simulink model "GFo_29bus"  (R2016b)
settings: Solver=ode1  StartTime=0.0  StopTime=4.5  FixedStep=Time_Step  RelTol=1e-3  EnableMultiTasking=on
PreLoadFcn:
  | Init_29bus;
InitFcn:
  | Init_29bus;
undefined symbols (not defined in the file): D1, D11, Delta, Time_Step, VSC01_Delta_P_Time_Step, VSC01_Delta_P_Value
libraries: powerlib x168, sps_avr x6, GFo_Lib x1
(part 1 of 4)
Description:
  | Copyright 2008-2017 The MathWorks, Inc.
settings Model: Creator=MathWorks  LastModifiedBy=Frederic_Colas
settings DataIOCC: SaveFormat=StructureWithTime  SignalLoggingSaveFormat=ModelDataLogs  SaveOutput=off  SignalLogging=off  DSMLogging=off  SaveTime=off
settings OptimizationCC: ExpressionDepthLimit=2147483647  LifeSpan=inf
settings DebuggingCC: UnderspecifiedInitializationDetection=Classic  MergeDetectMultiDrivingBlocksExec=none  SolverPrmCheckMsg=warning  FcnCallInpInsideContextMsg=warning  UnconnectedInputMsg=none  UnconnectedOutputMsg=none  UnconnectedLineMsg=none  StateNameClashWarn=warning  SFUnexpectedBacktrackingDiag=warning  SFNoUnconditionalDefaultTransitionDiag=warning  SFExecutionAtInitializationDiag=none
settings HardwareCC: ProdBitPerPointer=32  ProdBitPerSizeT=32  ProdBitPerPtrDiffT=32  ProdLargestAtomicFloat=None  ProdIntDivRoundTo=Undefined  ProdEndianess=Unspecified  ProdWordSize=32  ProdHWDeviceType=32-bit Generic
settings ModelReferenceCC: PropagateSignalLabelsOutOfModel=off
settings GRTTargetCC: TargetLangStandard=C89/C90 (ANSI)  GeneratePreprocessorConditionals=Disable all  CombineOutputUpdateFcns=off  GRTInterface=on
settings ConfigComp: CovMetricSettings=dw  CovHtmlReporting=on  CovSaveCumulativeToWorkspaceVar=on  CovSaveSingleToWorkspaceVar=on  CovExternalEMLEnable=off  CovSFcnEnable=off
settings SimscapeCC: SimscapeNormalizeSystem=off

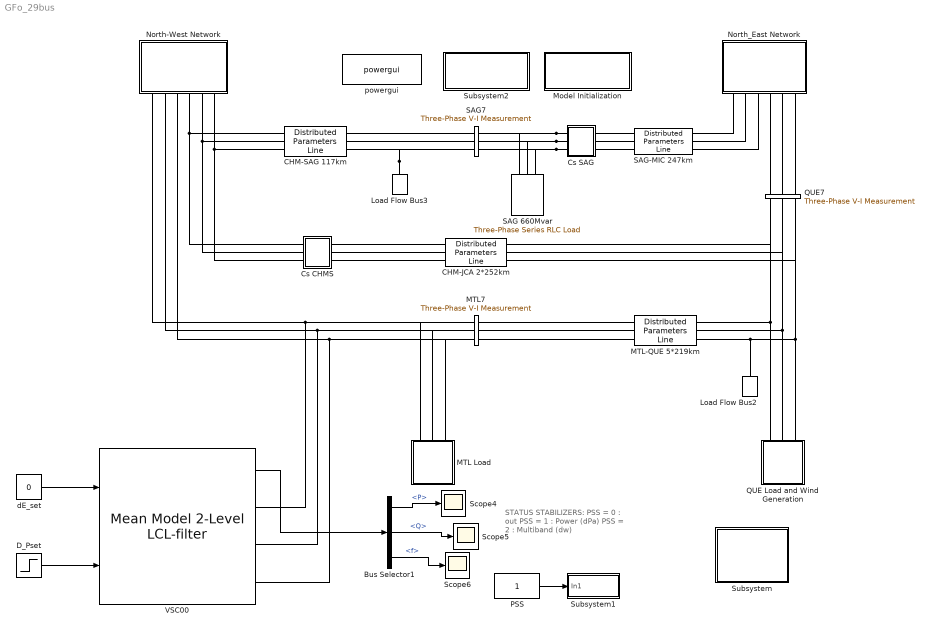
== system GFo_29bus ==
  note: STATUS STABILIZERS:
      | PSS = 0 :  out
      | PSS = 1 :  Power (dPa)
      | PSS = 2 :  Multiband (dw)
  Bus Selector1 : BusSelector  OutputSignals=control.P,control.Q,control.f
  CHM-JCA 2*252km : powerlib/Elements/Distributed Parameters Line  Phases=3  Frequency=60  Resistance="[0.01273  0.3864]/2"  Inductance="[0.9337e-3  4.1264e-3]/2"  Capacitance=[12.74e-9 7.751e-9]*2  Length=252  x1=[-0.00144 7.58185541586068e-08 0 0;-0.0014 7.65417383351047e-08 0 0;-0.00136 7.72475175803731e-08 0 0;-0.00132 7.7935731406298e-08 0 0;-0.00128 7.86062233189901e-08 0 0;-0.00124 7.92588408543707e-08 0 0;-0.0012 7.98934356128402e-08 0 0;-0.00116 8.0509863293023e-08 0 0;-0.00112 8.11079837245804e-08 0 0;-0.00108 8.16876609000843e-08 0 0;-0.00104 8.22487630059439e-08 0 0;-0.001 8.27911624523791e-08 0 0;-0.00096 8.33147359024331e-08 0 0;-0.00092 8.38193643000187e-08 0 0;-0.00088 8.43049328969899e-08 265107.476571619 -634085.697665156;-0.00084 8.4771331279235e-08 274638.71072506 -630016.083683103;-0.0008 8.52184533917841e-08 284107.494404066 -625803.209476646;-0.00076 8.56461975629245e-08 293511.674488884 -621448.033017052;-0.00072 8.60544665273205e-08 302849.112550059 -616951.54463389;-0.00068 8.64431674481302e-08 312117.6853347 -612314.766789841;-0.00064 8.68122119381164e-08 321315.285249284 -607538.753848202;-0.0006 8.71615160797445e-08 330439.820838908 -602624.591833129;-0.00056 8.7491000444265e-08 339489.217262864 -597573.398182686;-0.00052 8.78005901097747e-08 348461.416766445 -592386.32149475;-0.00048 8.80902146782535e-08 357354.379148857 -587064.541265828;-0.00044 8.83598082915721e-08 366166.082227143 -581609.267622851;-0.0004 8.86093096464677e-08 374894.522296013 -576021.741048002;-0.00036 8.88386620084838e-08 383537.714583465 -570303.232096638;-0.00032 8.90478132248713e-08 392093.693702109 -564455.041108381;-0.00028 8.9236715736447e-08 400560.514096078 -558478.497911428;-0.00024 8.94053265884089e-08 408936.250483427 -552374.961520165;-0.0002 8.95536074401033e-08 417218.998293933 -546145.81982613;-0.00016 8.96815245737432e-08 425406.87410217 -539792.489282428;-0.00012 8.97890489020757e-08 433498.016055789 -533316.414581635;-8e-05 8.98761559749955e-08 441490.584298885 -526719.068327291;-4e-05 8.99428259851056e-08 449382.761390363 -520001.950699042]  x2=[-0.00144 5.32803550600203e-08 0 0;-0.0014 5.36606177085858e-08 0 0;-0.00136 5.40286783954339e-08 0 0;-0.00132 5.43844534267383e-08 0 0;-0.00128 5.4727861902325e-08 0 0;-0.00124 5.50588257340681e-08 0 0;-0.0012 5.53772696636464e-08 0 0;-0.00116 5.56831212796564e-08 0 0;-0.00112 5.59763110340781e-08 0 0;-0.00108 5.62567722580899e-08 0 0;-0.00104 5.6524441177228e-08 0 0;-0.001 5.67792569258883e-08 0 0;-0.00096 5.70211615611672e-08 0 0;-0.00092 5.72501000760366e-08 0 0;-0.00088 5.74660204118525e-08 37391.1571539928 -657437.531518169;-0.00084 5.76688734701927e-08 47300.4110583682 -656799.004144863;-0.0008 5.78586131240209e-08 57198.9092571704 -656011.126342008;-0.00076 5.80351962281761e-08 67084.4009172698 -655074.077266222;-0.00072 5.81985826291833e-08 76954.6381631119 -653988.069994383;-0.00068 5.83487351743838e-08 86807.3765878642 -652753.351475181;-0.00064 5.84856197203837e-08 96640.3757637755 -651370.202472958;-0.0006 5.86092051408177e-08 106451.399751629 -649838.937503871;-0.00056 5.87194633334269e-08 116238.217609177 -648159.904764368;-0.00052 5.88163692264492e-08 125998.603898436 -646333.486052014;-0.00048 5.88999007843202e-08 135730.339191735 -644360.096678674;-0.00044 5.89700390126839e-08 145431.210576389 -642240.185376075;-0.0004 5.90267679627121e-08 155099.012157905 -639974.234193764;-0.00036 5.90700747347307e-08 164731.545561572 -637562.7583895;-0.00032 5.90999494811533e-08 174326.620432363 -635006.306312086;-0.00028 5.91163854087202e-08 183882.054932996 -632305.459276678;-0.00024 5.9119378780043e-08 193395.676240069 -629460.8314326;-0.0002 5.91089289144552e-08 202865.321038138 -626473.069623693;-0.00016 5.90850381881658e-08 212288.836011639 -623342.853241228;-0.00012 5.90477120337202e-08 221664.078334532 -620070.894069415;-8e-05 5.89969589387638e-08 230988.916157562 -616657.936123555;-4e-05 5.89327904441129e-08 240261.229093021 -613104.755480852]  x3=[-0.00144 2.36399872362907e-10 0 0;-0.0014 2.3698780301264e-10 0 0;-0.00136 2.37521844679663e-10 0 0;-0.00132 2.38001875927508e-10 0 0;-0.00128 2.38427787601207e-10 0 0;-0.00124 2.3879948285212e-10 0 0;-0.0012 2.39116877159951e-10 0 0;-0.00116 2.39379898351972e-10 0 0;-0.00112 2.39588486619432e-10 0 0;-0.00108 2.39742594531158e-10 0 0;-0.00104 2.3984218704434e-10 0 0;-0.001 2.39887241512498e-10 0 0;-0.00096 2.39877747690637e-10 0 0;-0.00092 2.39813707737568e-10 0 0;-0.00088 2.39695136215424e-10 455.571171588368 206.549514807623;-0.00084 2.39522060086348e-10 452.404295965122 213.395298242838;-0.0008 2.39294518706359e-10 449.134547506341 220.192557427475;-0.00076 2.39012563816404e-10 445.762669724628 226.939746723414;-0.00072 2.38676259530594e-10 442.289429355914 233.635331877992;-0.00068 2.38285682321623e-10 438.715616185106 240.277790372887;-0.00064 2.3784092100338e-10 435.0420428665 246.865611770318;-0.0006 2.37342076710754e-10 431.269544738988 253.397298056511;-0.00056 2.36789262876635e-10 427.398979636113 259.871363982331;-0.00052 2.36182605206121e-10 423.431227691001 266.286337401017;-0.00048 2.35522241647935e-10 419.367191136227 272.640759602933;-0.00044 2.34808322363056e-10 415.207794098658 278.93318564727;-0.0004 2.34041009690572e-10 410.95398238931 285.162184690607;-0.00036 2.33220478110768e-10 406.606723288283 291.32634031228;-0.00032 2.3234691420545e-10 402.167005324807 297.424250836457;-0.00028 2.31420516615516e-10 397.63583805246 303.454529650872;-0.00024 2.30441495995789e-10 393.014251819606 309.415805522124;-0.0002 2.29410074967115e-10 388.303297535099 315.306722907489;-0.00016 2.28326488065742e-10 383.504046429318 321.125942263154;-0.00012 2.27190981689987e-10 378.617589810576 326.872140348821;-8e-05 2.26003814044207e-10 373.64503881697 332.544010528597;-4e-05 2.24765255080087e-10 368.587524163715 338.140263068117]  x4=[-0.00144 2.98762369143109e-11 0 0;-0.0014 3.33610867134922e-11 0 0;-0.00136 3.68383504892487e-11 0 0;-0.00132 4.03072375417843e-11 0 0;-0.00128 4.37669590760978e-11 0 0;-0.00124 4.72167283813475e-11 0 0;-0.0012 5.0655761009743e-11 0 0;-0.00116 5.40832749549216e-11 0 0;-0.00112 5.74984908297697e-11 0 0;-0.00108 6.0900632043649e-11 0 0;-0.00104 6.42889249789862e-11 0 0;-0.001 6.76625991671874e-11 0 0;-0.00096 7.10208874638352e-11 0 0;-0.00092 7.43630262231319e-11 0 0;-0.00088 7.76882554715449e-11 191.292923698852 -10030.067654583;-0.00084 8.09958190806186e-11 342.515245147739 -10026.0432674796;-0.0008 8.42849649389116e-11 493.659681583605 -10019.7390445981;-0.00076 8.755494512302e-11 644.691864065019 -10011.1564194644;-0.00072 9.08050160676491e-11 795.57744917613 -10000.2973436934;-0.00068 9.40344387346936e-11 946.282126836066 -9987.16428654539;-0.00064 9.72424787812883e-11 1096.77162810075 -9971.76023436423;-0.0006 1.00428406726792e-10 1247.01173295536 -9954.08868989858;-0.00056 1.03591498118663e-10 1396.96827809566 -9934.15367150525;-0.00052 1.06731033697197e-10 1546.60716469647 -9911.95971223551;-0.00048 1.09846299559078e-10 1695.8943661654 -9887.51185880431;-0.00044 1.12936587319713e-10 1844.79593588023 -9860.81567044268;-0.0004 1.16001194274315e-10 1993.27801490809 -9831.87721763366;-0.00036 1.19039423557691e-10 2141.30683970465 -9800.70308073184;-0.00032 1.22050584302702e-10 2288.84874979171 -9767.30034846712;-0.00028 1.25033991797362e-10 2435.87019541126 -9731.67661633277;-0.00024 1.27988967640534e-10 2582.33774515442 -9693.83998485828;-0.0002 1.30914839896195e-10 2728.21809356346 -9653.79905776734;-0.00016 1.33810943246225e-10 2873.47806870518 -9611.56294002149;-0.00012 1.36676619141698e-10 3018.0846397139 -9567.14123574966;-8e-05 1.39511215952626e-10 3162.00492430239 -9520.54404606434;-4e-05 1.42314089116141e-10 3305.20619623907 -9471.78196676461]  x5=0.00142516474882927  V1=ones(3,3)  V2=ones(3,3)  I1=ones(3,3)  I2=ones(3,3)  nHarmo=1  Measurements=None
      settings: AttributesFormatString=\n
  CHM-SAG 117km : powerlib/Elements/Distributed Parameters Line  Phases=3  Frequency=60  Resistance="[0.01273  0.3864]"  Inductance="[0.9337e-3  4.1264e-3]"  Capacitance=[12.74e-9 7.751e-9]  Length=117  x1=[-0.00068 8.42693918023938e-08 0 0;-0.00064 8.46287304397579e-08 0 0;-0.0006 8.49688252336271e-08 0 0;-0.00056 8.52895988493781e-08 0 0;-0.00052 8.55909783458569e-08 0 0;-0.00048 8.5872895191965e-08 0 0;-0.00044 8.61352852822428e-08 290848.852660508 -619220.434969194;-0.0004 8.63780889514465e-08 300152.999076882 -614764.343999159;-0.00036 8.66012509881155e-08 309388.893289675 -610168.4609188;-0.00032 8.68047206471272e-08 318554.435136189 -605433.830792297;-0.00028 8.69884516612358e-08 327647.540451251 -600561.530233711;-0.00024 8.71524022515931e-08 336666.141541125 -595552.667162172;-0.0002 8.72965351372487e-08 345608.187653698 -590408.380549948;-0.00016 8.74208175436273e-08 354471.645444797 -585129.840163451;-0.00012 8.75252212099815e-08 363254.499440556 -579718.246297247;-8e-05 8.7609722395818e-08 371954.752495714 -574174.829501111;-4e-05 8.76743018862957e-08 380570.426247757 -568500.85030022]  x2=[-0.00068 5.85375290287409e-08 0 0;-0.00064 5.87422836781654e-08 0 0;-0.0006 5.89336808388534e-08 0 0;-0.00056 5.9111676988741e-08 0 0;-0.00052 5.92762316530388e-08 0 0;-0.00048 5.94273074134351e-08 0 0;-0.00044 5.95648699166049e-08 342746.554477027 -587488.694993711;-0.0004 5.96888878820212e-08 351566.310869505 -582253.6313362;-0.00036 5.97993331090682e-08 360306.12411467 -576886.168224064;-0.00032 5.98961804834537e-08 368964.006854359 -571387.526172128;-0.00028 5.99794079829199e-08 377537.9903607 -565758.955524177;-0.00024 6.00489966822511e-08 386026.124983782 -560001.736168637;-0.0002 6.01049307575773e-08 394426.480594989 -554117.177247541;-0.00016 6.01471974899721e-08 402737.147025899 -548106.616858843;-0.00012 6.0175787268345e-08 410956.234502632 -541971.421752141;-8e-05 6.0190693591627e-08 419081.874075575 -535712.987017895;-4e-05 6.01919130702487e-08 427112.218044361 -529332.735770193]  x3=[-0.00068 1.24684359191143e-10 0 0;-0.00064 1.23197676625095e-10 0 0;-0.0006 1.21682979969794e-10 0 0;-0.00056 1.20140613654197e-10 0 0;-0.00052 1.18570928399104e-10 0 0;-0.00048 1.16974281137405e-10 0 0;-0.00044 1.15351034932918e-10 1711.78655763124 -3591.74036566269;-0.0004 1.13701558897833e-10 1765.75158267616 -3565.52011206945;-0.00036 1.12026228108775e-10 1819.31509103836 -3538.48908995047;-0.00032 1.10325423521518e-10 1872.46490283797 -3510.65344592705;-0.00028 1.08599531884358e-10 1925.18893226613 -3482.01950958462;-0.00024 1.0684894565017e-10 1977.47519033321 -3452.59379203337;-0.0002 1.05074062887167e-10 2029.31178759503 -3422.38298442771;-0.00016 1.03275287188384e-10 2080.68693685638 -3391.39395644476;-0.00012 1.01453027579902e-10 2131.58895585138 -3359.63375472225;-8e-05 9.96076984278424e-11 2182.00626989986 -3327.10960125617;-4e-05 9.77397193441404e-11 2231.92741453938 -3293.82889175853]  x4=[-0.00068 5.36479088013724e-11 0 0;-0.00064 5.62282252514651e-11 0 0;-0.0006 5.87957558880272e-11 0 0;-0.00056 6.13499168767334e-11 0 0;-0.00052 6.38901274234009e-11 0 0;-0.00048 6.64158099060574e-11 0 0;-0.00044 6.89263900062868e-11 280.209360770516 -1025.16710784167;-0.0004 7.14212968398246e-11 295.636136449481 -1020.82529325836;-0.00036 7.38999630863721e-11 310.995687020474 -1016.25135180659;-0.00032 7.63618251185998e-11 326.284519854151 -1011.44632356119;-0.00028 7.88063231303119e-11 341.499158401772 -1006.41130114416;-0.00024 8.1232901263741e-11 356.636142985735 -1001.14742947617;-0.0002 8.36410077359454e-11 371.692031586282 -995.655905516244;-0.00016 8.603009496428e-11 386.663400624182 -989.937977989575;-0.00012 8.83996196909117e-11 401.546845739224 -983.994947103573;-8e-05 9.07490431063515e-11 416.338982564337 -977.828164252211;-4e-05 9.30778309719753e-11 431.036447495169 -971.439031708729]  x5=0.000661683633385019  V1=ones(3,3)  V2=ones(3,3)  I1=ones(3,3)  I2=ones(3,3)  nHarmo=1  Measurements=None
      settings: AttributesFormatString=\n
  Cs CHMS : Subsystem  mask{Xc=33/2}
      mask prompts: Xc "Condensator Reactance at  60Hz  (ohm):"
      mask help: Series Compensation
      mask init:
      | Cs=1/Xc/(2*pi*60);
      mask Display: disp('Cs')
  Cs SAG : Subsystem  mask{Xc=22}
      mask prompts: Xc "Condensator Reactance at  60Hz  (ohm):"
      mask help: Series Compensation
      mask init:
      | Cs=1/Xc/(2*pi*60);
      mask Display: disp('Cs')
  D_Pset : Step  Time=VSC01_Delta_P_Time_Step  After=VSC01_Delta_P_Value  SampleTime=0
  Load Flow Bus2 : powerlib/Measurements/Load Flow Bus  LConnTagsString=a  Phases=single  Connectors=on one side  ID=QUE7  Vbase=735e3  Vref=1  Vangle=0  VLF=1.016  VLFb=1  VLFc=1  angleLF=-12.43  angleLFb=0  angleLFc=0
      settings: AttributesFormatString=%<ID>\n%<Vbase>V\n%<VLF>pu\n%<angleLF>deg.
  Load Flow Bus3 : powerlib/Measurements/Load Flow Bus  LConnTagsString=a  Phases=single  Connectors=on one side  ID=SAG7  Vbase=735e3  Vref=1  Vangle=0  VLF=1.034  VLFb=1  VLFc=1  angleLF=2.23  angleLFb=0  angleLFc=0
      settings: AttributesFormatString=%<ID>\n%<Vbase>V\n%<VLF>pu\n%<angleLF>deg.
  MTL Load : Subsystem
  MTL-QUE 5*219km : powerlib/Elements/Distributed Parameters Line  Phases=3  Frequency=60  Resistance="[0.01273  0.3864]/5"  Inductance="[0.9337e-3  4.1264e-3]/5"  Capacitance=[12.74e-9 7.751e-9]*5  Length=219  x1=[-0.00124 3.13140205846512e-07 -185450.121801635 -635277.147887541;-0.0012 3.15795384732076e-07 -175849.670170163 -638001.383948039;-0.00116 3.18378754470456e-07 -166209.231840158 -640580.543995716;-0.00112 3.2088972762565e-07 -156530.99896416 -643014.041551821;-0.00108 3.23327733224018e-07 -146817.172288863 -645301.323259993;-0.00104 3.2569221688411e-07 -137069.960654684 -647441.869012097;-0.001 3.27982640942732e-07 -127291.580493494 -649435.192066489;-0.00096 3.30198484577206e-07 -117484.255324616 -651280.839158696;-0.00092 3.32339243923798e-07 -107650.215249218 -652978.390604485;-0.00088 3.34404432192293e-07 -97791.6964432079 -654527.460395296;-0.00084 3.36393579776688e-07 -87910.9406487465 -655927.696286018;-0.0008 3.38306234361977e-07 -78010.1946644932 -657178.779875083;-0.00076 3.40141961027001e-07 -68091.7098347044 -658280.426676874;-0.00072 3.41900342343347e-07 -58157.7415372972 -659232.386186407;-0.00068 3.43580978470266e-07 -48210.5486709954 -660034.441936299;-0.00064 3.45183487245598e-07 -38252.3931416758 -660686.411545989;-0.0006 3.46707504272665e-07 -28285.5393480304 -661188.146763211;-0.00056 3.4815268300314e-07 -18312.2536666614 -661539.533497702;-0.00052 3.4951869481584e-07 -8334.80393672679 -661740.49184715;-0.00048 3.50805229091459e-07 1644.54105574682 -661790.976115359;-0.00044 3.52011993283199e-07 11623.5120937662 -661690.974822642;-0.0004 3.53138712983289e-07 21599.8400453724 -661440.51070843;-0.00036 3.54185131985384e-07 31571.2563796214 -661039.640726103;-0.00032 3.55151012342829e-07 41535.4936824286 -660488.456030038;-0.00028 3.56036134422759e-07 51490.2861721592 -659787.081954881;-0.00024 3.56840296956046e-07 61433.3702148476 -658935.67798705;-0.0002 3.57563317083064e-07 71362.484838928 -657934.437728463;-0.00016 3.58205030395273e-07 81275.3722493598 -656783.588852522;-0.00012 3.58765290972599e-07 91169.7783410311 -655483.393052336;-8e-05 3.59243971416617e-07 101043.453211322 -654034.145981219;-4e-05 3.59640962879523e-07 110894.151671715 -652436.177185455]  x2=[-0.00124 5.50588257340681e-08 -51903.9427370369 -656450.777403812;-0.0012 5.53772696636464e-08 -41999.4092894903 -657158.855057256;-0.00116 5.56831212796564e-08 -32085.3255384587 -657717.500454157;-0.00112 5.59763110340782e-08 -22163.9458610917 -658126.586563369;-0.00108 5.62567722580899e-08 -12237.5262935698 -658386.020362239;-0.00104 5.6524441177228e-08 -2308.32401810053 -658495.742857757;-0.001 5.67792569258883e-08 7621.40315034427 -658455.729099975;-0.00096 5.70211615611672e-08 17549.3972774369 -658265.988187676;-0.00092 5.72501000760366e-08 27473.4008229281 -657926.563266307;-0.00088 5.74660204118525e-08 37391.1571539928 -657437.531518169;-0.00084 5.76688734701927e-08 47300.4110583682 -656799.004144863;-0.0008 5.78586131240209e-08 57198.9092571704 -656011.126342008;-0.00076 5.80351962281761e-08 67084.4009172698 -655074.077266222;-0.00072 5.81985826291833e-08 76954.6381631119 -653988.069994383;-0.00068 5.83487351743838e-08 86807.3765878643 -652753.351475181;-0.00064 5.84856197203837e-08 96640.3757637755 -651370.202472958;-0.0006 5.86092051408177e-08 106451.399751629 -649838.937503871;-0.00056 5.87194633334269e-08 116238.217609177 -648159.904764368;-0.00052 5.88163692264492e-08 125998.603898436 -646333.486052014;-0.00048 5.88999007843202e-08 135730.339191735 -644360.096678674;-0.00044 5.89700390126839e-08 145431.210576389 -642240.185376075;-0.0004 5.90267679627121e-08 155099.012157905 -639974.234193764;-0.00036 5.90700747347307e-08 164731.545561572 -637562.7583895;-0.00032 5.90999494811533e-08 174326.620432363 -635006.306312086;-0.00028 5.91163854087202e-08 183882.054932996 -632305.459276678;-0.00024 5.9119378780043e-08 193395.676240069 -629460.8314326;-0.0002 5.91089289144552e-08 202865.321038138 -626473.069623693;-0.00016 5.90850381881658e-08 212288.836011639 -623342.853241228;-0.00012 5.90477120337202e-08 221664.078334532 -620070.894069415;-8e-05 5.89969589387638e-08 230988.916157562 -616657.936123555;-4e-05 5.89327904441129e-08 240261.229093021 -613104.755480852]  x3=[-0.00124 2.99296411497035e-09 -6144.82838435572 -19926.8869416532;-0.0012 2.9563268208876e-09 -5843.65099570883 -20017.2814774563;-0.00116 2.91901728358006e-09 -5541.14481121902 -20103.1242560732;-0.00112 2.88104398691477e-09 -5237.37861818394 -20184.3957575961;-0.00108 2.84241556569193e-09 -4932.42149041631 -20261.0775015866;-0.00104 2.80314080368139e-09 -4626.34277253715 -20333.1520512774;-0.001 2.76322863162535e-09 -4319.2120642074 -20400.6030175373;-0.00096 2.72268812520754e-09 -4011.09920430154 -20463.4150625983;-0.00092 2.68152850298953e-09 -3702.07425502688 -20521.5739035431;-0.00088 2.63975912431445e-09 -3392.20748599195 -20575.0663155527;-0.00084 2.59738948717882e-09 -3081.56935822785 -20623.880134914;-0.0008 2.55442922607274e-09 -2770.23050816602 -20668.0042617853;-0.00076 2.51088810978911e-09 -2458.26173157608 -20707.4286627209;-0.00072 2.46677603920229e-09 -2145.73396746753 -20742.1443729517;-0.00068 2.42210304501672e-09 -1832.7182819588 -20772.1434984248;-0.00064 2.37687928548605e-09 -1519.28585211743 -20797.4192175977;-0.0006 2.33111504410318e-09 -1205.50794977506 -20817.9657829898;-0.00056 2.28482072726197e-09 -891.455925320772 -20833.7785224894;-0.00052 2.23800686189084e-09 -577.201191476651 -20844.8538404158;-0.00048 2.19068409305906e-09 -262.81520705916 -20851.1892183372;-0.00044 2.14286318155617e-09 51.6305392699954 -20852.7832156434;-0.0004 2.09455500144507e-09 366.064545259763 -20849.6354698731;-0.00036 2.0457705375893e-09 680.415311328745 -20841.7466967966;-0.00032 1.99652088315527e-09 994.611356823582 -20829.1186902527;-0.00028 1.94681723708966e-09 1308.58123627304 -20811.7543217414;-0.00024 1.89667090157298e-09 1622.25355563409 -20789.6575397702;-0.0002 1.84609327944948e-09 1935.55698852632 -20762.8333689569;-0.00016 1.79509587163426e-09 2248.42029245088 -20731.2879088865;-0.00012 1.74369027449807e-09 2560.77232499049 -20695.0283327246;-8e-05 1.69188817723041e-09 2872.54205998656 -20654.0628855862;-4e-05 1.63970135918147e-09 3183.65860368993 -20608.4008826607]  x4=[-0.00124 -9.87973508675663e-10 -1607.24957615672 -3120.54597153218;-0.0012 -9.24127780471541e-10 -1560.01251794718 -3144.42715530081;-0.00116 -8.60071913579479e-10 -1512.42072634402 -3167.59332345071;-0.00112 -7.95820473751212e-10 -1464.48502331026 -3190.03920819502;-0.00108 -7.31388071210079e-10 -1416.21630901138 -3211.75970553312;-0.00104 -6.66789357328774e-10 -1367.62555933676 -3232.74987641121;-0.001 -6.0203902129776e-10 -1318.72382340385 -3253.00494784545;-0.00096 -5.37151786785065e-10 -1269.52222104568 -3272.52031400727;-0.00092 -4.72142408588256e-10 -1220.03194028234 -3291.29153727071;-0.00088 -4.07025669279315e-10 -1170.26423477689 -3309.31434922145;-0.00084 -3.41816375843222e-10 -1120.23042127638 -3326.58465162749;-0.0008 -2.7652935631096e-10 -1069.94187703853 -3343.098517371;-0.00076 -2.1117945638776e-10 -1019.41003724462 -3358.85219134131;-0.00072 -1.45781536077312e-10 -968.646392399267 -3373.84209128882;-0.00068 -8.03504663027266e-11 -917.662485717529 -3388.06480863955;-0.00064 -1.49011255250167e-11 -866.469910500123 -3401.51710927021;-0.0006 5.05516036401357e-11 -815.080307497187 -3414.19593424366;-0.00056 1.15992837806559e-10 -763.50536226128 -3426.09840050444;-0.00052 1.81407696201944e-10 -711.756802490185 -3437.22180153436;-0.00048 2.46781304051607e-10 -659.846395360132 -3447.56360796794;-0.00044 3.1209879596088e-10 -607.785944850047 -3457.1214681676;-0.0004 3.77345319295376e-10 -555.587289057427 -3465.89320875834;-0.00036 4.42506037558352e-10 -503.262297506455 -3473.876835122;-0.00032 5.07566133764397e-10 -450.82286844898 -3481.07053185079;-0.00028 5.72510813808688e-10 -398.28092615895 -3487.47266316011;-0.00024 6.37325309831042e-10 -345.64841822094 -3493.08177326051;-0.0002 7.01994883573999e-10 -292.937312813372 -3497.89658668873;-0.00016 7.66504829734178e-10 -240.159595987053 -3501.91600859771;-0.00012 8.30840479306131e-10 -187.327268939656 -3505.13912500557;-8e-05 8.94987202917954e-10 -134.452345286743 -3507.56520300344;-4e-05 9.58930414157873e-10 -81.5468483299793 -3509.1936909221]  x5=0.00123853603172068  V1=ones(3,3)  V2=ones(3,3)  I1=ones(3,3)  I2=ones(3,3)  nHarmo=1  Measurements=None
      settings: AttributesFormatString=\n
  MTL7 : powerlib/Measurements/Three-Phase V-I Measurement  VoltageMeasurement=phase-to-ground  SetLabelV=on  LabelV=Vabc_MTL7  Vpu=on  VpuLL=off  CurrentMeasurement=no  SetLabelI=off  LabelI=A1  Ipu=off  Pbase=100e6  Vbase=735e3  OutputType=Magnitude  PhasorSimulation=off  PSBequivalent=0
  Model Initialization : Subsystem  mask(Model Functions){InitFcnX=Init_29bus;, prel=on, posl=off, inif=on, strf=off}
      mask prompts: InitFcnX "Initialisation"; prel "Preload Function"; posl "PostLoad Function"; inif "InitFcn"; strf "StartFcn"
      mask init:
      | currentBlock = gcb;
      | root = bdroot(currentBlock);
      | 
      | if ~strcmp(get_param(root,'BlockDiagramType'),'library')
      |     if prel==1
      |         set_param(root, 'PreLoadFcn', InitFcnX);
      |     else
      |         set_param(root, 'PreLoadFcn', '');
      |     end
      |     if inif==1
      |         set_param(root, 'InitFcn', InitFcnX);
      |     else
      |         set_param(root, 'InitFcn', '');
      |     end
      |     if strf==1
      |         set_param(root, 'StartFcn', InitFcnX);
      |     else
      |         set_param(root, 'StartFcn', '');
      |     end
      |     if posl==1
      |         set_param(root, 'PostLoadFcn', InitFcnX);
      |     else
      |         set_param(root, 'PostLoadFcn', '');
      |     end
      | end
      | 
      | pos = get_param(currentBlock, 'Position');
      | width = pos(3) - pos(1); height = pos(4) - pos(2);
      | txt = [ upper(root) '\n' '- InitFcn. . . . . '  get_param(root, 'InitFcn') ];
      settings: CopyFcn=set_param(gcb,'LinkStatus','none')
      mask Display:
      | %text(5, height*0.5, txt, 'horizontalAlignment', 'left', 'verticalAlignment', 'middle') ;
      | color('blue'),disp('Initialization Function\nParameters')
  North-West Network : Subsystem
  North_East Network : Subsystem
  PSS : Constant
  QUE Load and Wind Generation : Subsystem
  QUE7 : powerlib/Measurements/Three-Phase V-I Measurement  VoltageMeasurement=no  SetLabelV=on  LabelV=Vabc_QUE7  Vpu=on  VpuLL=off  CurrentMeasurement=no  SetLabelI=off  LabelI=A1  Ipu=off  Pbase=100e6  Vbase=735e3  OutputType=Magnitude  PhasorSimulation=off  PSBequivalent=0
  SAG 660Mvar : powerlib/Elements/Three-Phase Series RLC Load  LConnTagsString=A|B|C  Configuration=Y (grounded)  NominalVoltage=735e3  Vabc=[1e3 1e3 1e3]  Vabcp=[1e3 1e3 1e3]  NominalFrequency=60  UnbalancedPower=off  ActivePower=2200000  InductivePower=660e6  CapacitivePower=0  Pabc=[10e3 9e3 11e3]  QLabc=[100 90 110]  QCabc=[100 90 110]  Pabcp=[10e3 9e3 11e3]  QLabcp=[100 90 110]  QCabcp=[100 90 110]  Measurements=None  LoadType=constant Z
  SAG-MIC 247km : powerlib/Elements/Distributed Parameters Line  Phases=3  Frequency=60  Resistance="[0.01273  0.3864]/1"  Inductance="[0.9337e-3  4.1264e-3]/1"  Capacitance=[12.74e-9 7.751e-9]*1  Length=247  x1=[-0.0014 5.40873341776019e-08 78356.1362806858 -664124.955272439;-0.00136 5.45312309755495e-08 88361.5766055067 -662867.963935626;-0.00132 5.49627278418306e-08 98346.9242698054 -661460.242140145;-0.00128 5.53817266577788e-08 108309.908691633 -659902.10998979;-0.00124 5.57881321466767e-08 118248.264374249 -658193.921790378;-0.0012 5.61818518954209e-08 128159.731421276 -656336.065969173;-0.00116 5.65627963755356e-08 138042.056050579 -654328.964986568;-0.00112 5.69308789635314e-08 147892.991106762 -652173.075240017;-0.00108 5.72860159606018e-08 157710.296572141 -649868.886960258;-0.00104 5.76281266116564e-08 167491.740076115 -647416.924099835;-0.001 5.79571331236833e-08 177235.097402784 -644817.744213957;-0.00096 5.82729606834388e-08 186938.152996713 -642071.938333716;-0.00092 5.85755374744596e-08 196598.700466737 -639180.130831691;-0.00088 5.88647946933926e-08 206214.54308767 -636142.97927997;-0.00084 5.91406665656407e-08 215783.494299823 -632961.174300623;-0.0008 5.94030903603191e-08 225303.378206209 -629635.439408666;-0.00076 5.96520064045201e-08 234772.030067326 -626166.530847531;-0.00072 5.98873580968816e-08 244187.296793393 -622555.237417112;-0.00068 6.01090919204585e-08 253547.03743395 -618802.380294393;-0.00064 6.03171574548914e-08 262849.123664692 -614908.812846718;-0.0006 6.05115073878721e-08 272091.440271427 -610875.42043775;-0.00056 6.06920975259018e-08 281271.88563106 -606703.12022614;-0.00052 6.08588868043405e-08 290388.372189486 -602392.860956975;-0.00048 6.10118372967446e-08 299438.82693628 -597945.622746043;-0.00044 6.1150914223491e-08 308421.191876078 -593362.416856963;-0.0004 6.12760859596861e-08 317333.424496555 -588644.285471228;-0.00036 6.13873240423563e-08 326173.498232868 -583792.30145123;-0.00032 6.14846031769211e-08 334939.402928484 -578807.568096292;-0.00028 6.15679012429441e-08 343629.145292267 -573691.218891793;-0.00024 6.16371992991634e-08 352240.749351744 -568444.41725142;-0.0002 6.16924815877987e-08 360772.256902412 -563068.35625262;-0.00016 6.17337355381341e-08 369221.727953028 -557564.258365303;-0.00012 6.17609517693773e-08 377587.24116674 -551933.375173863;-8e-05 6.17741240927919e-08 385866.894297985 -546176.987092579;-4e-05 6.17732495131051e-08 394058.80462504 -540296.40307446]  x2=[-0.0014 1.88321190355134e-08 207429.358640792 -660594.51265032;-0.00136 1.89772310245538e-08 217366.870028888 -657391.600759257;-0.00132 1.9118027754912e-08 227254.95406523 -654039.203687286;-0.00128 1.92544772106255e-08 237091.362284782 -650538.08374059;-0.00124 1.93865483642649e-08 246873.857973139 -646889.037043652;-0.0012 1.95142111839887e-08 256600.216675142 -643092.893358225;-0.00116 1.96374366403727e-08 266268.226700699 -639150.515894644;-0.00112 1.97561967130107e-08 275875.689627704 -635062.801115549;-0.00108 1.98704643968863e-08 285420.420801939 -630830.678532028;-0.00104 1.99802137085137e-08 294900.249833843 -626455.110492261;-0.001 2.00854196918458e-08 304313.021092047 -621937.091962687;-0.00096 2.01860584239492e-08 313656.594193539 -617277.650301758;-0.00092 2.02821070204442e-08 322928.84449037 -612477.845026326;-0.00088 2.03735436407082e-08 332127.663552784 -607538.767570718;-0.00084 2.04603474928422e-08 341250.959648653 -602461.541038557;-0.0008 2.05424988383989e-08 350296.65821912 -597247.31994737;-0.00076 2.06199789968707e-08 359262.702350339 -591897.289966069;-0.00072 2.06927703499377e-08 368147.053241192 -586412.667645334;-0.00068 2.0760856345474e-08 376947.690666903 -580794.700140985;-0.00064 2.08242215013114e-08 385662.613438416 -575044.664930383;-0.0006 2.08828514087598e-08 394289.839857445 -569163.86952195;-0.00056 2.09367327358838e-08 402827.408167101 -563153.651157848;-0.00052 2.09858532305345e-08 411273.376997975 -557015.376509903;-0.00048 2.10302017231348e-08 419625.825809591 -550750.441368836;-0.00044 2.106976812922e-08 427882.855327117 -544360.270326871;-0.0004 2.11045434517305e-08 436042.587973246 -537846.316453797;-0.00036 2.1134519783058e-08 444103.168295141 -531210.06096655;-0.00032 2.11596903068431e-08 452062.763386348 -524453.0128924;-0.00028 2.11800492995259e-08 459919.563303584 -517576.708725808;-0.00024 2.11955921316469e-08 467671.781478303 -510582.712079043;-0.0002 2.12063152689001e-08 475317.655122943 -503472.61332663;-0.00016 2.12122162729367e-08 482855.445631773 -496248.029243709;-0.00012 2.12132938019192e-08 490283.438976234 -488910.602638398;-8e-05 2.12095476108268e-08 497599.946094697 -481462.001978234;-4e-05 2.12009785515111e-08 504803.303276536 -473903.92101077]  x3=[-0.0014 8.54566736572813e-11 -14.0413794849774 -3976.64390507056;-0.00136 8.48160555079537e-11 45.9239992686561 -3976.40393558055;-0.00132 8.4156150919026e-11 105.878935300888 -3975.25976612663;-0.00128 8.34771099471111e-11 165.809795376294 -3973.21165688308;-0.00124 8.27790870002702e-11 225.702951734113 -3970.26007357226;-0.0012 8.20622408029018e-11 285.544785187088 -3966.40568735879;-0.00116 8.13267343596495e-11 345.321688218344 -3961.64937469683;-0.00112 8.05727349183357e-11 405.020068075627 -3955.99221713087;-0.00108 7.98004139319312e-11 464.626349862174 -3949.43550104977;-0.00104 7.90099470195679e-11 524.126979623529 -3941.98071739421;-0.001 7.82015139266052e-11 583.508427429597 -3933.6295613177;-0.00096 7.73752984837567e-11 642.757190451229 -3924.38393180113;-0.00092 7.65314885652892e-11 701.859796030655 -3914.24593122091;-0.00088 7.56702760463014e-11 760.802804745044 -3903.21786487095;-0.00084 7.47918567590933e-11 819.572813462519 -3891.30224043844;-0.0008 7.38964304486357e-11 878.156458389907 -3878.50176743361;-0.00076 7.29842007271497e-11 936.540418111556 -3864.81935657365;-0.00072 7.20553750278073e-11 994.711416618506 -3850.25811912078;-0.00068 7.11101645575627e-11 1052.65622632734 -3834.82136617484;-0.00064 7.01487842491257e-11 1110.36167108804 -3818.51260792031;-0.0006 6.91714527120877e-11 1167.81462918007 -3801.3355528282;-0.00056 6.81783921832123e-11 1225.00203629624 -3783.2941068127;-0.00052 6.71698284758997e-11 1281.91088851332 -3764.39237234304;-0.00048 6.61459909288397e-11 1338.52824524908 -3744.63464751065;-0.00044 6.51071123538612e-11 1394.84123220485 -3724.02542505177;-0.0004 6.40534289829933e-11 1450.83704429301 -3702.56939132587;-0.00036 6.29851804147478e-11 1506.50294854879 -3680.27142524997;-0.00032 6.19026095596371e-11 1561.82628702559 -3657.13659718928;-0.00028 6.0805962584938e-11 1616.79447967334 -3633.17016780419;-0.00024 5.96954888587153e-11 1671.39502719905 -3608.37758685407;-0.0002 5.85714408931181e-11 1725.61551390908 -3582.76449195802;-0.00016 5.74340742869604e-11 1779.44361053232 -3556.33670731295;-0.00012 5.62836476676002e-11 1832.86707702379 -3529.10024236917;-8e-05 5.51204226321299e-11 1885.87376534792 -3501.06129046395;-4e-05 5.39446636878913e-11 1938.45162224089 -3472.22622741314]  x4=[-0.0014 -8.38683564651098e-12 272.469707999068 -1043.89342109225;-0.00136 -6.659437897953e-12 288.179694547293 -1039.66611261533;-0.00132 -4.93052585064556e-12 303.824151518133 -1035.2023930301;-0.00128 -3.20049264427872e-12 319.399521496986 -1030.5032773479;-0.00124 -1.46973167348446e-12 334.902262779035 -1025.56983410711;-0.0012 2.61363501617935e-13 350.328850174602 -1020.40318513018;-0.00116 1.99239924491395e-12 365.675775810746 -1015.00450526853;-0.00112 3.7229819338034e-12 380.939549928925 -1009.37502213542;-0.00108 5.45271804870673e-12 396.116701678532 -1003.51601582675;-0.00104 7.18121426254803e-12 411.203779906143 -997.428818630033;-0.001 8.90807753019417e-12 426.197353940274 -991.114814721421;-0.00096 1.06329151778299e-11 441.094014371488 -984.575439850952;-0.00092 1.23553349922486e-11 455.890373827666 -977.812181016077;-0.00088 1.4074945310038e-11 470.583067744268 -970.826576123532;-0.00084 1.57913551066409e-11 485.1687551294 -963.620213639629;-0.0008 1.75041740852715e-11 499.644119323532 -956.19473222905;-0.00076 1.92130127656646e-11 514.005868753678 -948.551820382235;-0.00072 2.09174825726408e-11 528.250737681867 -940.693216031428;-0.00068 2.26171959244647e-11 542.375486947748 -932.620706155488;-0.00064 2.43117663209778e-11 556.376904705143 -924.336126373546;-0.0006 2.60008084314852e-11 570.251807152399 -915.841360527603;-0.00056 2.76839381823766e-11 583.997039256351 -907.138340254155;-0.00052 2.93607728444616e-11 597.609475469751 -898.229044544961;-0.00048 3.10309311199982e-11 611.086020441995 -889.115499297035;-0.00044 3.26940332293975e-11 624.423609722971 -879.799776851974;-0.0004 3.43497009975818e-11 637.619210459896 -870.283995524728;-0.00036 3.59975579399784e-11 650.669822086956 -860.570319121908;-0.00032 3.76372293481292e-11 663.572477007612 -850.660956449763;-0.00028 3.92683423748958e-11 676.324241269401 -840.558160811908;-0.00024 4.08905261192422e-11 688.922215231097 -830.26422949695;-0.0002 4.25034117105739e-11 701.363534222062 -819.781503256098;-0.00016 4.41066323926165e-11 713.645369193647 -809.1123657709;-0.00012 4.56998236068124e-11 725.764927362492 -798.259243111214;-8e-05 4.72826230752186e-11 737.719452845585 -787.224603183539;-4e-05 4.88546708828854e-11 749.506227286923 -776.010955169835]  x5=0.00139688767047948  V1=ones(3,3)  V2=ones(3,3)  I1=ones(3,3)  I2=ones(3,3)  nHarmo=1  Measurements=None
      settings: AttributesFormatString=\n
  SAG7 : powerlib/Measurements/Three-Phase V-I Measurement  VoltageMeasurement=no  SetLabelV=on  LabelV=Vabc_SAG7  Vpu=on  VpuLL=off  CurrentMeasurement=no  SetLabelI=off  LabelI=Iabc_SAG7  Ipu=off  Pbase=100e6  Vbase=735e3  OutputType=Magnitude  PhasorSimulation=off  PSBequivalent=0
  Scope4 : Scope
  Scope5 : Scope
  Scope6 : Scope
  Subsystem : Subsystem
      mask Display: disp('Display\nWaveforms')
  Subsystem1 : Subsystem
      mask Display: disp('PSS_select')
  Subsystem2 : Subsystem
      settings: OpenFcn=LoadFlow_VSC
      mask Display: color('blue'),disp('Update Loadflow')
  VSC00 : GFo_Lib/Mean Model 2-Level LCL-filter  fn=50  Sn=VSC01_Sn  Pn=VSC01_Pn  Udcn=640e3  Un1=VSC01_Un1  Un2=VSC01_Un2  Rt_pu=VSC01_Rt_pu  Lt_pu=VSC01_Lt_pu  Rm_pu=500  Lm_pu=0  Lf_pu=VSC01_Lf_pu  Rf_pu=VSC01_Rf_pu  Cf_pu=VSC01_Cf_pu  Tr_PLL=VSC01_Tr_PLL  Val_Freq_Support=on  Val_gamma=on  R_percent=VSC01_R  Rv=VSC01_Rv  W_TVR=VSC01_W_LF  I_thresh_pu=1  DX_DR=5  Kp_Rvi_pu=0.676  gainpopup=3  wc1=VSC01_wc1  mp1=VSC01_mp1  wc2=VSC01_wc2  mp2=VSC01_mp2  wc3=VSC01_wc3  mp3=VSC01_mp3  T1=VSC01_T1  T2=VSC01_T2  LFpopup=PV  P0=0.9  Q0=-0.23678  V0=1  Theta0=-20.9713  innercontrol=1  Kp_i=0.73  Ki_i=1.19  Kp_v=0.52  Ki_v=1.16  Kffv=1  Kffi=1  I_max=1.25
  dE_set : Constant  Value=0
  powergui : powerlib/powergui  Priority=1  SimulationMode=Discrete  SampleTime=Time_Step  frequency=60  Iterations=50  frequencyindice=60  Pbase=1e+008  ErrMax=0.0001  UnitsV=kV  UnitsW=MW  buscounter=0  FunctionMessages=off  echomessages=off  EnableUseOfTLC=off  CurrentSourceSwitches=off  DisableSnubberDevices=off  DisableRonSwitches=off  DisableVfSwitches=off  DisplayEquations=off  SolverType=Tustin/Backward Euler (TBE)  Interpol=off  ExternalGateDelay=off  methode=off  Ts=100  x0status=blocks  SPID=off  SwTol=0  HookPort=off  RestoreLinks=warning  ResistiveCurrentMeasurement=off  Frange=[0:2:500]  Ylog=off  Xlog=on  ShowGrid=off  save=off  variable=ZData  structure=0  ZoomFFT=off  StartTime=0.0  cycles=1  DisplayStyle=1  fundamental=60  FreqAxis=off  MaxFrequency=1000  frequencyindicesteady=1  RmsSteady=1  display=off
  wires:
  PSS/1 -> Subsystem1/1(In1)
  D_Pset/1 -> VSC00/2
  dE_set/1 -> VSC00/1
  Bus Selector1/3 -> Scope6/1  "<f>"
  Bus Selector1/2 -> Scope5/1  "<Q>"
  VSC00/1 -> Bus Selector1/1
  Bus Selector1/1 -> Scope4/1  "<P>"
  connections:
  QUE Load and Wind Generation/LConn3 -- MTL-QUE 5*219km/RConn3 -- Load Flow Bus2/LConn1 -- CHM-JCA 2*252km/RConn3 -- QUE7/LConn3
  MTL7/RConn1 -- MTL-QUE 5*219km/LConn1
  MTL7/RConn2 -- MTL-QUE 5*219km/LConn2
  MTL7/RConn3 -- MTL-QUE 5*219km/LConn3
  QUE Load and Wind Generation/LConn2 -- MTL-QUE 5*219km/RConn2 -- CHM-JCA 2*252km/RConn2 -- QUE7/LConn2
  QUE Load and Wind Generation/LConn1 -- MTL-QUE 5*219km/RConn1 -- CHM-JCA 2*252km/RConn1 -- QUE7/LConn1
  Cs SAG/LConn1 -- SAG7/RConn1 -- SAG 660Mvar/LConn1
  Cs SAG/LConn2 -- SAG7/RConn2 -- SAG 660Mvar/LConn2
  Cs SAG/LConn3 -- SAG7/RConn3 -- SAG 660Mvar/LConn3
  Load Flow Bus3/LConn1 -- CHM-SAG 117km/RConn3 -- SAG7/LConn3
  Cs CHMS/LConn1 -- CHM-SAG 117km/LConn1 -- North-West Network/RConn4
  Cs CHMS/LConn2 -- CHM-SAG 117km/LConn2 -- North-West Network/RConn5
  Cs CHMS/LConn3 -- CHM-SAG 117km/LConn3 -- North-West Network/RConn6
  Cs SAG/RConn1 -- SAG-MIC 247km/LConn1
  Cs SAG/RConn3 -- SAG-MIC 247km/LConn3
  Cs CHMS/RConn3 -- CHM-JCA 2*252km/LConn3
  Cs CHMS/RConn2 -- CHM-JCA 2*252km/LConn2
  Cs CHMS/RConn1 -- CHM-JCA 2*252km/LConn1
  Cs SAG/RConn2 -- SAG-MIC 247km/LConn2
  SAG7/LConn2 -- CHM-SAG 117km/RConn2
  SAG7/LConn1 -- CHM-SAG 117km/RConn1
  SAG-MIC 247km/RConn1 -- North_East Network/LConn1
  SAG-MIC 247km/RConn2 -- North_East Network/LConn2
  SAG-MIC 247km/RConn3 -- North_East Network/LConn3
  QUE7/RConn1 -- North_East Network/LConn4
  QUE7/RConn2 -- North_East Network/LConn5
  QUE7/RConn3 -- North_East Network/LConn6
  MTL7/LConn1 -- MTL Load/LConn1 -- VSC00/RConn1 -- North-West Network/RConn1
  MTL7/LConn2 -- MTL Load/LConn2 -- VSC00/RConn2 -- North-West Network/RConn2
  MTL7/LConn3 -- MTL Load/LConn3 -- VSC00/RConn3 -- North-West Network/RConn3

== system GFo_29bus/Cs CHMS ==
  note: B
  Ca : powerlib/Elements/Series RLC Branch  LConnTagsString=__new0  RConnTagsString=__new0  BranchType=C  Resistance=1.0  Inductance=1.0  SetiL0=off  InitialCurrent=0  Capacitance=Cs  Setx0=off  InitialVoltage=0  Measurements=None
  Cb : powerlib/Elements/Series RLC Branch  LConnTagsString=__new0  RConnTagsString=__new0  BranchType=C  Resistance=1.0  Inductance=1.0  SetiL0=off  InitialCurrent=0  Capacitance=Cs  Setx0=off  InitialVoltage=0  Measurements=None
  Cc : powerlib/Elements/Series RLC Branch  LConnTagsString=__new0  RConnTagsString=__new0  BranchType=C  Resistance=1.0  Inductance=1.0  SetiL0=off  InitialCurrent=0  Capacitance=Cs  Setx0=off  InitialVoltage=0  Measurements=None
  A : PMIOPort  Port=1  Side=Left
  B : PMIOPort  Port=2  Side=Left
  C : PMIOPort  Port=3  Side=Left
  "A " : PMIOPort  Port=4  Side=Right
  "B " : PMIOPort  Port=5  Side=Right
  "C " : PMIOPort  Port=6  Side=Right
  connections:
  Cc/RConn1 -- "C "/RConn1
  C/RConn1 -- Cc/LConn1
  Cb/RConn1 -- "B "/RConn1
  B/RConn1 -- Cb/LConn1
  Ca/RConn1 -- "A "/RConn1
  A/RConn1 -- Ca/LConn1

== system GFo_29bus/Cs SAG ==
  note: B
  Ca : powerlib/Elements/Series RLC Branch  LConnTagsString=__new0  RConnTagsString=__new0  BranchType=C  Resistance=1.0  Inductance=1.0  SetiL0=off  InitialCurrent=0  Capacitance=Cs  Setx0=off  InitialVoltage=0  Measurements=None
  Cb : powerlib/Elements/Series RLC Branch  LConnTagsString=__new0  RConnTagsString=__new0  BranchType=C  Resistance=1.0  Inductance=1.0  SetiL0=off  InitialCurrent=0  Capacitance=Cs  Setx0=off  InitialVoltage=0  Measurements=None
  Cc : powerlib/Elements/Series RLC Branch  LConnTagsString=__new0  RConnTagsString=__new0  BranchType=C  Resistance=1.0  Inductance=1.0  SetiL0=off  InitialCurrent=0  Capacitance=Cs  Setx0=off  InitialVoltage=0  Measurements=None
  A : PMIOPort  Port=1  Side=Left
  B : PMIOPort  Port=2  Side=Left
  C : PMIOPort  Port=3  Side=Left
  "A " : PMIOPort  Port=4  Side=Right
  "B " : PMIOPort  Port=5  Side=Right
  "C " : PMIOPort  Port=6  Side=Right
  connections:
  A/RConn1 -- Ca/LConn1
  Ca/RConn1 -- "A "/RConn1
  B/RConn1 -- Cb/LConn1
  Cb/RConn1 -- "B "/RConn1
  C/RConn1 -- Cc/LConn1
  Cc/RConn1 -- "C "/RConn1

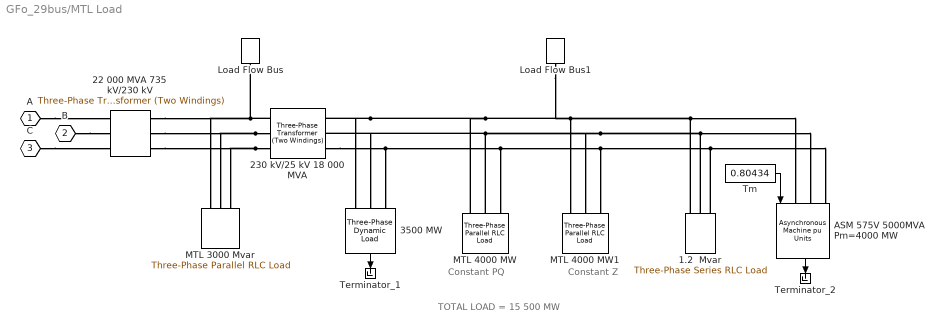
== system GFo_29bus/MTL Load ==
  note: Constant PQ
  note: Constant Z
  note: TOTAL LOAD = 15 500 MW
  1.2  Mvar : powerlib/Elements/Three-Phase Series RLC Load  LConnTagsString=A|B|C  Configuration=Y (grounded)  NominalVoltage=25e3  Vabc=[1e3 1e3 1e3]  Vabcp=[1e3 1e3 1e3]  NominalFrequency=60  UnbalancedPower=off  ActivePower=2000e6/50  InductivePower=0  CapacitivePower=2000e6  Pabc=[10e3 9e3 11e3]  QLabc=[100 90 110]  QCabc=[100 90 110]  Pabcp=[10e3 9e3 11e3]  QLabcp=[100 90 110]  QCabcp=[100 90 110]  Measurements=None  LoadType=constant Z
  22 000 MVA 735 kV/230 kV : powerlib/Elements/Three-Phase Transformer (Two Windings)  Winding1Connection=Yg  Winding2Connection=Delta (D1)  CoreType=Three single-phase transformers  SetSaturation=off  Hysteresis=off  DataFile='basic_model'  SetInitialFlux=off  Measurements=None  UNITS=pu  NominalPower=[ 22000e6 60 ]  Winding1="[ 735e3 0.002  0.12]"  Winding2=[230e3 0.002 0]  Rm=500  Lm=500  L0=0.5  Saturation="[ 0,0  ;  0.005,1.2  ;  1.0,1.4 ]"  InitialFluxes=[ 0.8 , -0.8 , 0.7 ]  MoreParameters=off  BreakLoop=off  DataType=off  TransfoNumber=0
  230 kV/25 kV 18 000 MVA : powerlib/Elements/Three-Phase Transformer (Two Windings)  Winding1Connection=Yg  Winding2Connection=Delta (D1)  CoreType=Three single-phase transformers  SetSaturation=off  Hysteresis=off  DataFile='basic_model'  SetInitialFlux=off  Measurements=None  UNITS=pu  NominalPower=[18000e6 60 ]  Winding1="[ 230e3  0.08/30   0.08 ]"  Winding2="[ 25e3  0.08/30  0.08]"  Rm=500  Lm=500  L0=0.5  Saturation="[ 0,0  ;  0.005,1.2  ;  1.0,1.4 ]"  InitialFluxes=[ 0.8 , -0.8 , 0.7 ]  MoreParameters=off  BreakLoop=off  DataType=off  TransfoNumber=0
  3500 MW : powerlib/Elements/Three-Phase Dynamic Load  NominalVoltage=[ 25e3 60 ]  ActiveReactivePowers=[3.5e+09 4.44089e-08]  PositiveSequence=[0.977579 -93.983]  ExternalControl=off  NpNq="[1.5  2.5]"  TimeConstants="[0  0  0  0]"  MinimumVoltage=0.7  Tfilter=1e-4  LoadFlowParameters=[4,0,0,0,0]
  ASM 575V 5000MVA Pm=4000 MW : powerlib/Machines/Asynchronous Machine pu Units  RotorType=Squirrel-cage  PresetModel=No  MechanicalLoad=Torque Tm  ShowDetailedParameters=on  ReferenceFrame=Rotor  Units=pu  MeasurementBus=off  NominalParameters="[5000e6 25e3  60]"  Stator=[0.01117 0.04832]  Rotor=[0.006 0.04832]  Cage1=[0.01909 0.0397]  Cage2=[0.01909 0.0397]  Lm=2.424  Mechanical="[1  0   2]"  PolePairs=2  InitialConditions=[0.00539423 0 0.951058 0.951058 0.951058 -122.82 -242.82 -2.82009]  SimulateSaturation=off  Saturation="[0.212,0.4201,0.8125,1.0979,1.4799,2.2457,3.2586,4.5763,6.4763 ;   0.5,0.7,0.9,1,1.1,1.2 ,1.3,1.4,1.5]"  LoadFlowParameters=0  TsPowergui=0  TsBlock=-1  IterativeModel=Trapezoidal non iterative  IterativeDiscreteModel=Trapezoidal non iterative  Pmec=4000000000
  Load Flow Bus : powerlib/Measurements/Load Flow Bus  LConnTagsString=a  Phases=single  Connectors=on one side  ID=MTL2  Vbase=230e3  Vref=1  Vangle=0  VLF=0.9954  VLFb=1  VLFc=1  angleLF=-55.87  angleLFb=0  angleLFc=0
      settings: AttributesFormatString=%<ID>\n%<Vbase>V\n%<VLF>pu\n%<angleLF>deg.
  Load Flow Bus1 : powerlib/Measurements/Load Flow Bus  LConnTagsString=a  Phases=single  Connectors=on one side  ID=MTL_25  Vbase=25e3  Vref=1  Vangle=0  VLF=0.9776  VLFb=1  VLFc=1  angleLF=-93.98  angleLFb=0  angleLFc=0
      settings: AttributesFormatString=%<ID>\n%<Vbase>V\n%<VLF>pu\n%<angleLF>deg.
  MTL 3000 Mvar : powerlib/Elements/Three-Phase Parallel RLC Load  LConnTagsString=A|B|C  Configuration=Y (grounded)  NominalVoltage=230e3  Vabc=[1e3 1e3 1e3]  Vabcp=[1e3 1e3 1e3]  NominalFrequency=60  UnbalancedPower=off  ActivePower=0  InductivePower=0  CapacitivePower=3000e6  Pabc=[10e3 9e3 11e3]  QLabc=[100 90 110]  QCabc=[100 90 110]  Pabcp=[10e3 9e3 11e3]  QLabcp=[100 90 110]  QCabcp=[100 90 110]  Measurements=None  LoadType=constant Z
  MTL 4000 MW : powerlib/Elements/Three-Phase Parallel RLC Load  LConnTagsString=A|B|C  Configuration=Y (grounded)  NominalVoltage=(25000)*0.977579  Vabc=[1e3 1e3 1e3]  Vabcp=[1e3 1e3 1e3]  NominalFrequency=60  UnbalancedPower=off  ActivePower=4000000000  InductivePower=0  CapacitivePower=0  Pabc=[10e3 9e3 11e3]  QLabc=[100 90 110]  QCabc=[100 90 110]  Pabcp=[10e3 9e3 11e3]  QLabcp=[100 90 110]  QCabcp=[100 90 110]  Measurements=None  LoadType=constant PQ
  MTL 4000 MW1 : powerlib/Elements/Three-Phase Parallel RLC Load  LConnTagsString=A|B|C  Configuration=Y (grounded)  NominalVoltage=25e3  Vabc=[1e3 1e3 1e3]  Vabcp=[1e3 1e3 1e3]  NominalFrequency=60  UnbalancedPower=off  ActivePower=4000000000  InductivePower=0  CapacitivePower=0  Pabc=[10e3 9e3 11e3]  QLabc=[100 90 110]  QCabc=[100 90 110]  Pabcp=[10e3 9e3 11e3]  QLabcp=[100 90 110]  QCabcp=[100 90 110]  Measurements=None  LoadType=constant Z
  Terminator_1 : Terminator
  Terminator_2 : Terminator
  Tm : Constant  Value=0.80434
  A : PMIOPort  Port=1  Side=Left
  B : PMIOPort  Port=2  Side=Left
  C : PMIOPort  Port=3  Side=Left
  wires:
  Tm/1 -> ASM 575V 5000MVA Pm=4000 MW/1
  3500 MW/1 -> Terminator_1/1
  ASM 575V 5000MVA Pm=4000 MW/1 -> Terminator_2/1
  connections:
  A/RConn1 -- 22 000 MVA 735 kV/230 kV/LConn1
  B/RConn1 -- 22 000 MVA 735 kV/230 kV/LConn2
  C/RConn1 -- 22 000 MVA 735 kV/230 kV/LConn3
  230 kV/25 kV 18 000 MVA/LConn1 -- Load Flow Bus/LConn1 -- 22 000 MVA 735 kV/230 kV/RConn1 -- MTL 3000 Mvar/LConn1
  230 kV/25 kV 18 000 MVA/LConn2 -- 22 000 MVA 735 kV/230 kV/RConn2 -- MTL 3000 Mvar/LConn2
  230 kV/25 kV 18 000 MVA/LConn3 -- 22 000 MVA 735 kV/230 kV/RConn3 -- MTL 3000 Mvar/LConn3
  MTL 4000 MW1/LConn1 -- Load Flow Bus1/LConn1 -- MTL 4000 MW/LConn1 -- 230 kV/25 kV 18 000 MVA/RConn1 -- 3500 MW/LConn1 -- ASM 575V 5000MVA Pm=4000 MW/LConn1 -- 1.2  Mvar/LConn1
  MTL 4000 MW1/LConn2 -- MTL 4000 MW/LConn2 -- 230 kV/25 kV 18 000 MVA/RConn2 -- 3500 MW/LConn2 -- ASM 575V 5000MVA Pm=4000 MW/LConn2 -- 1.2  Mvar/LConn2
  230 kV/25 kV 18 000 MVA/RConn3 -- ASM 575V 5000MVA Pm=4000 MW/LConn3 -- 1.2  Mvar/LConn3 -- MTL 4000 MW1/LConn3 -- MTL 4000 MW/LConn3 -- 3500 MW/LConn3

== system GFo_29bus/Model Initialization ==
